simulink model "questao1"  (R2021b)
settings: Solver=VariableStepAuto  StartTime=0.0  StopTime=1800  RelTol=1e-3
values from neighbouring files (symbols this model uses):
  dF = 0    [main.m]
  dFj = 4.72e-5    (= 4.72e-05)    [main.m]
  dTi = 0    [main.m]
  dTij = 0    [main.m]
  Fjs = 7.079e-4    (= 0.0007079)    [main.m]
  Fs = 4.720e-4    (= 0.000472)    [main.m]
  Tis = 10    [main.m]
  Tjis = 93.33    [main.m]
  Tjs = 65.56    [main.m]
  Ts = 51.67    [main.m]
settings Model: Creator=luang  LastModifiedBy=luang

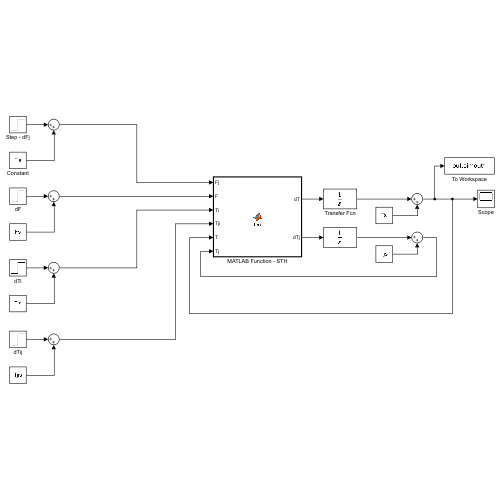
[thumbnail: Simulink's stored preview of the top-level diagram]
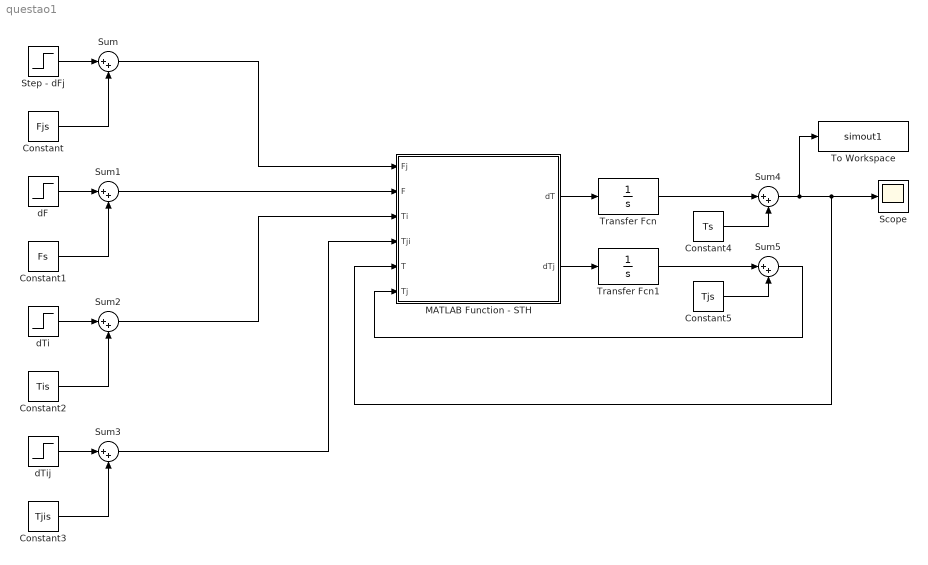
== system questao1 ==
  Constant : Constant  Value=Fjs
  Constant1 : Constant  Value=Fs
  Constant2 : Constant  Value=Tis
  Constant3 : Constant  Value=Tjis
  Constant4 : Constant  Value=Ts
  Constant5 : Constant  Value=Tjs
  MATLAB Function - STH : MATLAB Function  TreatAsAtomicUnit=on
  Scope : Scope
  Step - dFj : Step  After=dFj  SampleTime=0
  Sum{,1..5} (6 alike) : Sum  Inputs=|++
  To Workspace : ToWorkspace  VariableName=simout1  SaveFormat=Structure With Time  SampleTime=-1
  Transfer Fcn : TransferFcn  Denominator=[1 0]
  Transfer Fcn1 : TransferFcn  Denominator=[1 0]
  dF : Step  After=dF  SampleTime=0
  dTi : Step  After=dTi  SampleTime=0
  dTij : Step  After=dTij  SampleTime=0
  wires:
  Step - dFj/1 -> Sum/1
  Constant/1 -> Sum/2
  Constant1/1 -> Sum1/2
  dF/1 -> Sum1/1
  Constant2/1 -> Sum2/2
  dTi/1 -> Sum2/1
  Constant3/1 -> Sum3/2
  dTij/1 -> Sum3/1
  Sum/1 -> MATLAB Function - STH/1(Fj)
  Sum1/1 -> MATLAB Function - STH/2(F)
  Sum2/1 -> MATLAB Function - STH/3(Ti)
  Sum3/1 -> MATLAB Function - STH/4(Tji)
  MATLAB Function - STH/1(dT) -> Transfer Fcn/1
  MATLAB Function - STH/2(dTj) -> Transfer Fcn1/1
  Transfer Fcn/1 -> Sum4/1
  Constant4/1 -> Sum4/2
  Constant5/1 -> Sum5/2
  Transfer Fcn1/1 -> Sum5/1
  Sum4/1 -> To Workspace/1, MATLAB Function - STH/5(T), Scope/1
  Sum5/1 -> MATLAB Function - STH/6(Tj)

== matlab function questao1/MATLAB Function - STH ==
  data: Fj input; dT output; F input; Ti input; Tji input; T input; Tj input; dTj output
function [dT, dTj] = fcn(Fj, F, Ti, Tji, T, Tj)

V = 283.168e-3;
UA = 3.065;
pcp = 2.165e3;
Vj = 28.319e-3;
pcpj = 2.165e3;

dT = (F/V)*(Ti - T) + (UA/(V*pcp))*(Tj - T);

dTj = (Fj/Vj)*(Tji - Tj) - ((UA/(Vj*pcpj))*(Tj - T));
